simulink model "Binay_MN_SIMULINK_No8"  (R2023b)
settings: Solver=VariableStepAuto  StartTime=0.0  StopTime=20  RelTol=1e-3
settings Model: Creator=ninabinay  LastModifiedBy=ninabinay

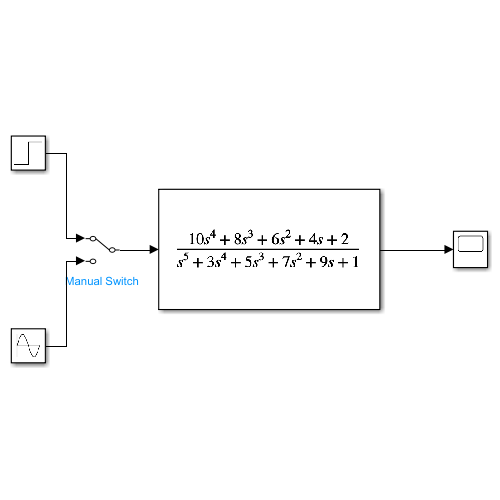
[thumbnail: Simulink's stored preview of the top-level diagram]
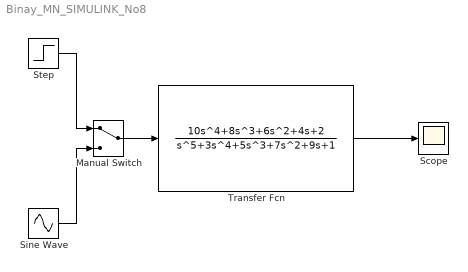
== system Binay_MN_SIMULINK_No8 ==
  Manual Switch : ManualSwitch
  Scope : Scope
  Sine Wave : Sin  SampleTime=0
  Step : Step  Time=0  SampleTime=0
  Transfer Fcn : TransferFcn  Numerator=[10 8 6 4 2]  Denominator=[1 3 5 7 9 1]
  wires:
  Transfer Fcn/1 -> Scope/1
  Step/1 -> Manual Switch/1
  Sine Wave/1 -> Manual Switch/2
  Manual Switch/1 -> Transfer Fcn/1
